simulink model "consensus"  (Simulink 7.8)
settings: Solver=ode45  StartTime=0.0  StopTime=10.0  RelTol=1e-3
settings Model: Creator=chepeadan  LastModifiedBy=Tigervilla
settings DebuggingCC: FcnCallInpInsideContextMsg=Use local settings  StrictBusMsg=Warning

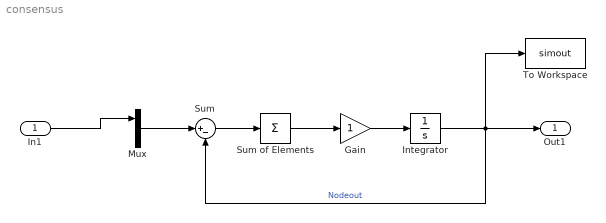
== system consensus ==
  In1 : Inport
  Gain : Gain
  Integrator : Integrator  InitialCondition=100*(rand()-0.5)
  Mux : Mux  Inputs=2
  Sum : Sum  Inputs=|+-
  Sum of Elements : Sum  Inputs=+
  To Workspace : ToWorkspace  VariableName=simout  SampleTime=-1  SaveFormat=Structure With Time
  Out1 : Outport
  wires:
  In1/1 -> Mux/1
  Mux/1 -> Sum/1
  Sum/1 -> Sum of Elements/1
  Sum of Elements/1 -> Gain/1
  Gain/1 -> Integrator/1
  Integrator/1 -> Out1/1, Sum/2, To Workspace/1  "Nodeout"
